simulink model "JGVD_Non_Isothermal_CSTR"  (R2022a)
settings: Solver=VariableStepAuto  StartTime=0.0  StopTime=200  RelTol=1e-3
values from neighbouring files (symbols this model uses):
  seedPI = 3    [JGVD_Mixing_Tank_Parameters.m]    (also in JGVD_Non_Isothermal_CSTR_Parameters.m)
  varPI = 5E-5    (= 5e-05)    [JGVD_Mixing_Tank_Parameters.m]    (also in JGVD_Non_Isothermal_CSTR_Parameters.m)
undefined symbols (not defined in the file or in its folder): p
settings Model: Creator=georg  LastModifiedBy=georg

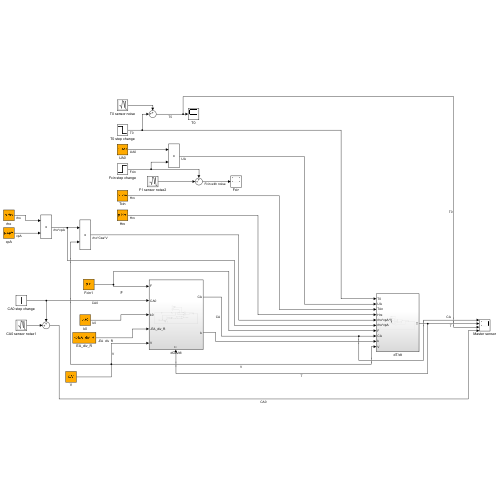
[thumbnail: Simulink's stored preview of the top-level diagram]
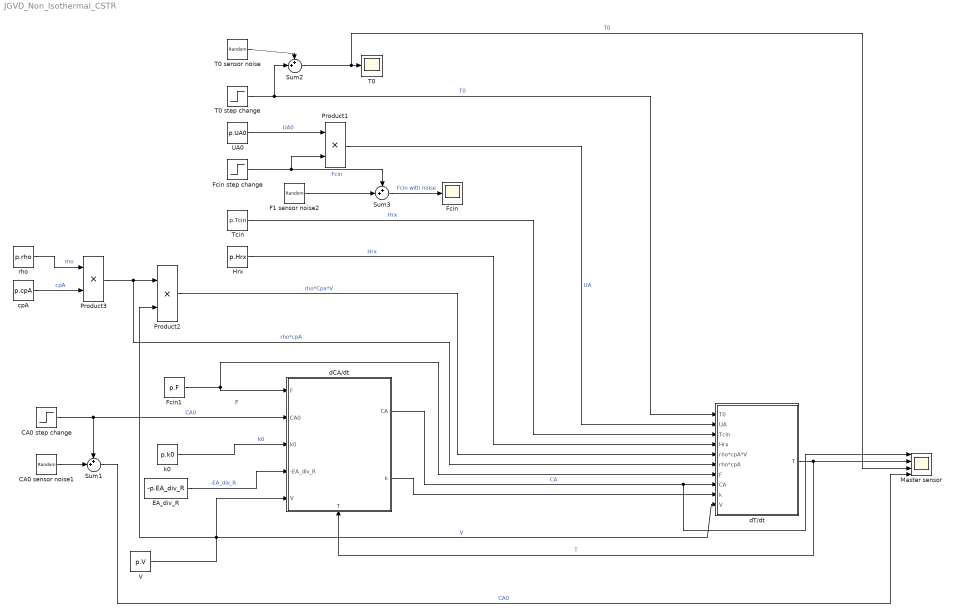
== system JGVD_Non_Isothermal_CSTR ==
  note: F
  CA0 sensor noise1 : RandomNumber  Variance=varPI  Seed=seedPI  SampleTime=0.1
  CA0 step change : Step  Time=20  Before=p.CA0  After=p.CA0  SampleTime=0
  EA_div_R : Constant  Value=-p.EA_div_R
  F1 sensor noise2 : RandomNumber  Variance=varPI  Seed=seedPI  SampleTime=0.1
  Fcin : Scope
  Fcin step change : Step  Time=20  Before=p.Fcin  After=p.Fcin  SampleTime=0
  Fcin1 : Constant  Value=p.F
  Hrx : Constant  Value=p.Hrx
  Master sensor : Scope  NumInputPorts=4
  Product1 : Product
  Product2 : Product
  Product3 : Product
  Sum1 : Sum  Inputs=++|
  Sum2 : Sum  Inputs=++|
  Sum3 : Sum  Inputs=++|
  T0 : Scope
  T0 sensor noise : RandomNumber  Variance=varPI  Seed=seedPI  SampleTime=0.1
  T0 step change : Step  Time=20  Before=p.T0  After=p.T0*0.9  SampleTime=0
  Tcin : Constant  Value=p.Tcin
  UA0 : Constant  Value=p.UA0
  V : Constant  Value=p.V
  cpA : Constant  Value=p.cpA
  dCA/dt : Subsystem
      settings: PortSchema="{\"entries\":[{\"content\":{\"sides\":[{\"content\":{\"connectorIds\":[\"In1\",\"In2\",\"In3\",\"In4\",\"In5\"]},\"type\":\"ConnectorPlacement.EquallySpacedRectSide\",\"uuid\":\"0f4bfc8b-2ae4-4dd4-bd66-74fe07ca36d4\"},{\"content\":{\"connectorIds\":[\"Out1\",\"Out2\"],\"side\":\"RIGHT\"},\"type\":\"ConnectorPlacement.EquallySpacedRectSide\",\"uuid\":\"52c9f69f-1c31-420b-afe7-2c8a65db04f5\"},{\"content\":{\"connectorIds\":[],\"side\":\"TOP\"},\"type\":\"ConnectorPlacement.EquallySpacedRectSide\",\"uuid\":\"eda348c0-49da-4438-86b7-5a4db3f9afc7\"},{\"content\":{\"connectorIds\":[\"In6\"],\"side\":\"BOTTOM\"},\"type\":\"ConnectorPlacement.EquallySpacedRectSide\",\"uuid\":\"72a3153b-a3c9-473a-8a15-955ee2e27a15\"}]},\"type\":\"ConnectorPlacement.EquallySpacedConnector\",\"uuid\":\"848d482c-2eb5-4d08-af25-ae63985b7c38\"}],\"packageUris\":[\"http://schema.mathworks.com/mf0/Connector/R2020b\"],\"version\":\"1.0\"}"
  dT/dt : Subsystem
  k0 : Constant  Value=p.k0
  rho : Constant  Value=p.rho
  wires:
  Product1/1 -> dT/dt/2(UA)  "UA"
  UA0/1 -> Product1/1  "UA0"
  Fcin step change/1 -> Sum3/1, Product1/2  "Fcin"
  dCA/dt/1(CA) -> Master sensor/1, dT/dt/8(CA)  "CA"
  Fcin1/1 -> dCA/dt/1(F), dT/dt/7(F)
  V/1 -> Product2/2, dCA/dt/5(V), dT/dt/10(V)  "V"
  k0/1 -> dCA/dt/3(k0)  "k0"
  EA_div_R/1 -> dCA/dt/4(-EA_div_R)  "-EA_div_R"
  Hrx/1 -> dT/dt/4(Hrx)  "Hrx"
  T0 step change/1 -> dT/dt/1(T0), Sum2/2  "T0"
  dCA/dt/2(k) -> dT/dt/9(k)
  rho/1 -> Product3/1  "rho"
  cpA/1 -> Product3/2  "cpA"
  Product2/1 -> dT/dt/5(rho*cpA*V)  "rho*Cpa*V"
  Product3/1 -> dT/dt/6(rho*cpA), Product2/1  "rho*cpA"
  dT/dt/1(T) -> dCA/dt/6(T), Master sensor/2  "T"
  Tcin/1 -> dT/dt/3(Tcin)  "Hrx"
  CA0 step change/1 -> dCA/dt/2(CA0), Sum1/1  "CA0"
  T0 sensor noise/1 -> Sum2/1
  CA0 sensor noise1/1 -> Sum1/2
  F1 sensor noise2/1 -> Sum3/2
  Sum2/1 -> Master sensor/3, T0/1  "T0"
  Sum3/1 -> Fcin/1  "Fcin with noise"
  Sum1/1 -> Master sensor/4  "CA0"

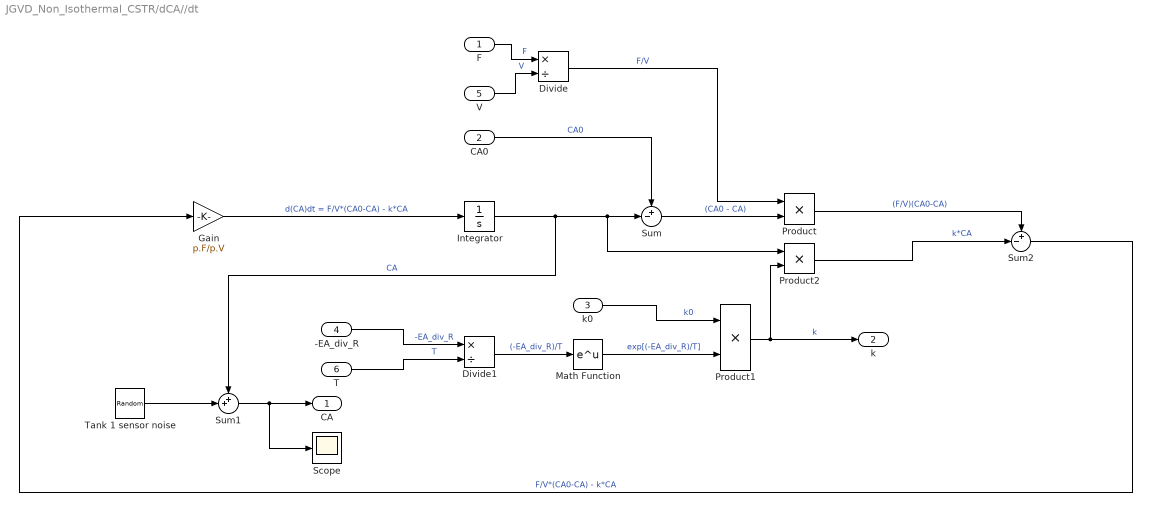
== system JGVD_Non_Isothermal_CSTR/dCA//dt ==
  F : Inport
  CA0 : Inport  Port=2
  k0 : Inport  Port=3
  -EA_div_R : Inport  Port=4
  V : Inport  Port=5
  T : Inport  Port=6
  Divide : Product  Inputs=*/
  Divide1 : Product  Inputs=*/
  Gain : Gain  Gain=p.F/p.V
  Integrator : Integrator  InitialCondition=p.CAs
  Math Function : Math
  Product : Product
  Product1 : Product
  Product2 : Product
  Scope : Scope
  Sum : Sum  Inputs=+-|
  Sum1 : Sum  Inputs=++|
  Sum2 : Sum  Inputs=+-|
  Tank 1 sensor noise : RandomNumber  Variance=0  SampleTime=0.1
  CA : Outport
  k : Outport  Port=2
  wires:
  Sum1/1 -> Scope/1, CA/1
  CA0/1 -> Sum/1  "CA0"
  Gain/1 -> Integrator/1  "d(CA)dt = F/V*(CA0-CA) - k*CA"
  Integrator/1 -> Product2/1, Sum/2, Sum1/1  "CA"
  Product/1 -> Sum2/1  "(F/V)(CA0-CA)"
  Sum/1 -> Product/2  "(CA0 - CA)"
  Tank 1 sensor noise/1 -> Sum1/2
  F/1 -> Divide/1  "F"
  V/1 -> Divide/2  "V"
  Divide/1 -> Product/1  "F/V"
  Divide1/1 -> Math Function/1  "(-EA_div_R)/T"
  Product1/1 -> k/1, Product2/2  "k"
  k0/1 -> Product1/1  "k0"
  Math Function/1 -> Product1/2  "exp[(-EA_div_R)/T]"
  -EA_div_R/1 -> Divide1/1  "-EA_div_R"
  T/1 -> Divide1/2  "T"
  Product2/1 -> Sum2/2  "k*CA"
  Sum2/1 -> Gain/1  "F/V*(CA0-CA) - k*CA"

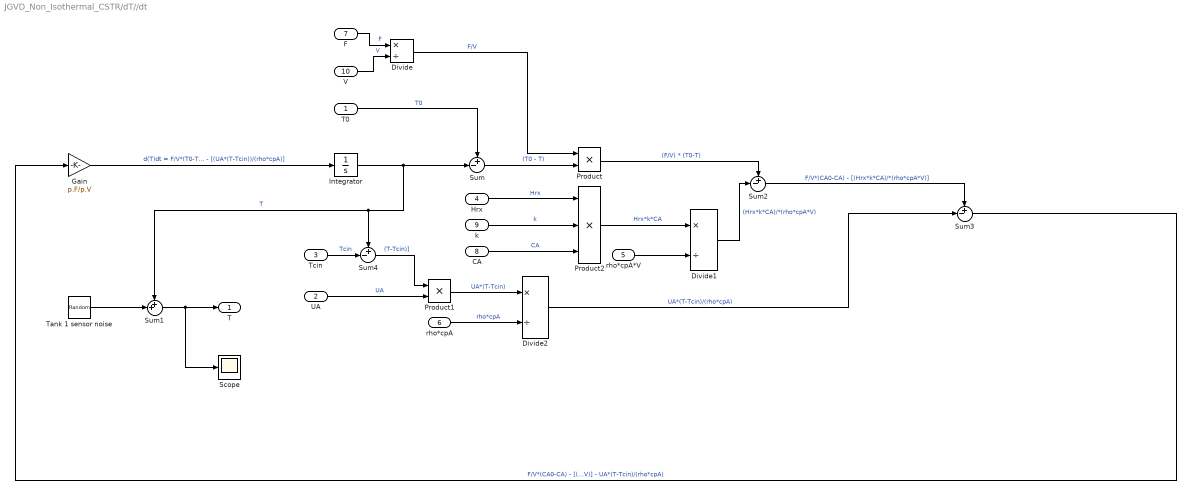
== system JGVD_Non_Isothermal_CSTR/dT//dt ==
  T0 : Inport
  UA : Inport  Port=2
  Tcin : Inport  Port=3
  Hrx : Inport  Port=4
  rho*cpA*V : Inport  Port=5
  rho*cpA : Inport  Port=6
  F : Inport  Port=7
  CA : Inport  Port=8
  k : Inport  Port=9
  V : Inport  Port=10
  Divide : Product  Inputs=*/
  Divide1 : Product  Inputs=*/
  Divide2 : Product  Inputs=*/
  Gain : Gain  Gain=p.F/p.V
  Integrator : Integrator  InitialCondition=p.Ts
  Product : Product
  Product1 : Product
  Product2 : Product  Inputs=3
  Scope : Scope
  Sum{,2..4} (4 alike) : Sum  Inputs=+-|
  Sum1 : Sum  Inputs=++|
  Tank 1 sensor noise : RandomNumber  Variance=0.00005  SampleTime=0.1
  T : Outport
  wires:
  CA/1 -> Product2/3  "CA"
  Product2/1 -> Divide1/1  "Hrx*k*CA"
  F/1 -> Divide/1  "F"
  Gain/1 -> Integrator/1  "d(T)dt = F/V*(T0-T) - [(Hrx*k*CA)/(rho*cpA*V)] - [(UA*(T-Tcin))/(rho*cpA)]"
  Integrator/1 -> Sum/2, Sum4/1, Sum1/1  "T"
  Sum1/1 -> Scope/1, T/1
  k/1 -> Product2/2  "k"
  Tank 1 sensor noise/1 -> Sum1/2
  Divide/1 -> Product/1  "F/V"
  Sum/1 -> Product/2  "(T0 - T)"
  Sum2/1 -> Sum3/1  "F/V*(CA0-CA) - [(Hrx*k*CA)/*(rho*cpA*V)]"
  T0/1 -> Sum/1  "T0"
  V/1 -> Divide/2  "V"
  Product/1 -> Sum2/1  "(F/V) * (T0-T)"
  Hrx/1 -> Product2/1  "Hrx"
  rho*cpA*V/1 -> Divide1/2
  Divide1/1 -> Sum2/2  "(Hrx*k*CA)/*(rho*cpA*V)"
  Tcin/1 -> Sum4/2  "Tcin"
  Sum4/1 -> Product1/1  "(T-Tcin)]"
  UA/1 -> Product1/2  "UA"
  Product1/1 -> Divide2/1  "UA*(T-Tcin)"
  rho*cpA/1 -> Divide2/2  "rho*cpA"
  Divide2/1 -> Sum3/2  "UA*(T-Tcin)/(rho*cpA)"
  Sum3/1 -> Gain/1  "F/V*(CA0-CA) - [(Hrx*k*CA)/*(rho*cpA*V)] - UA*(T-Tcin)/(rho*cpA)"
